simulink model "simulinkDEC"  (R2013b)
settings: Solver=ode45  StartTime=0.0  StopTime=10.0  RelTol=1e-3
undefined symbols (not defined in the file or in its folder): dfilt
libraries: dspsigops x4, dsparch4 x4, dspsrcs4 x1
settings Model: Creator=Johan  LastModifiedBy=Johan

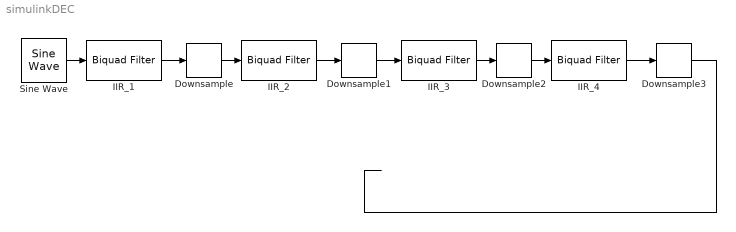
== system simulinkDEC ==
  Downsample{,1..3} (4 alike) : dspsigops/Downsample  N=2  phase=0  RateOptions=Enforce single-rate processing  smode=Allow multirate  fmode=Maintain input frame size  ic=0
  IIR_1 : dsparch4/Biquad Filter  Tag=BlockMethodSubSystem  IIRFiltStruct=Direct form I  CoeffSource=Specify via dialog  BiQuadCoeffs=[1 2 1 1 -1.70675000346131567 0.76497690612845648]  a0Flag=None  IC=0  ICnum=0  ICden=0  denAccumFracLength=30  denProdOutputFracLength=30  secondMemoryFracLength=15  roundingMode=Floor  overflowMode=off  ScaleValues=[0.014556725666785229;1]  optimizeScaleValues=off  ScaleValueMode=Specify via input port (g)  scaleValueFracLength=14  FilterSource=Specify via dialog  dfiltObjectName=dfilt.df2tsos([1 0.3 0.4],[1 0.1 0.2])
  IIR_2 : dsparch4/Biquad Filter  Tag=BlockMethodSubSystem  IIRFiltStruct=Direct form I  CoeffSource=Specify via dialog  BiQuadCoeffs=[1 2 1 1 -1.60151276454445912 0.700754075354693917]  a0Flag=Warning  IC=0  ICnum=0  ICden=0  denAccumFracLength=30  denProdOutputFracLength=30  secondMemoryFracLength=15  roundingMode=Floor  overflowMode=off  ScaleValues=[0.0248103277025586919;0.891250938133745563]  optimizeScaleValues=on  ScaleValueMode=Specify via input port (g)  scaleValueFracLength=14  FilterSource=Specify via dialog  dfiltObjectName=dfilt.df2tsos([1 0.3 0.4],[1 0.1 0.2])
  IIR_3 : dsparch4/Biquad Filter  Tag=BlockMethodSubSystem  IIRFiltStruct=Direct form I  CoeffSource=Specify via dialog  BiQuadCoeffs=[1 2 1 1 -1.29699998625984003 0.553258028437339289]  a0Flag=Warning  IC=0  ICnum=0  ICden=0  denAccumFracLength=30  denProdOutputFracLength=30  secondMemoryFracLength=15  roundingMode=Floor  overflowMode=off  ScaleValues=[0.0640645105443748281;0.891250938133745563]  optimizeScaleValues=on  ScaleValueMode=Specify via input port (g)  scaleValueFracLength=14  FilterSource=Specify via dialog  dfiltObjectName=dfilt.df2tsos([1 0.3 0.4],[1 0.1 0.2])
  IIR_4 : dsparch4/Biquad Filter  Tag=BlockMethodSubSystem  IIRFiltStruct=Direct form I  CoeffSource=Specify via dialog  BiQuadCoeffs=[1 2 1 1 -0.720403563238159794 0.382932497160983876]  a0Flag=Warning  IC=0  ICnum=0  ICden=0  denAccumFracLength=30  denProdOutputFracLength=30  secondMemoryFracLength=15  roundingMode=Floor  overflowMode=off  ScaleValues=[0.165632233480706048;0.891250938133745563]  optimizeScaleValues=on  ScaleValueMode=Specify via input port (g)  scaleValueFracLength=14  FilterSource=Specify via dialog  dfiltObjectName=dfilt.df2tsos([1 0.3 0.4],[1 0.1 0.2])
  Sine Wave : dspsrcs4/Sine Wave  Amplitude=5  Frequency=20000  Phase=0  SampleMode=Discrete  OutComplex=Real  CompMethod=Trigonometric fcn  TableSize=Speed  SampleTime=1/768000  SamplesPerFrame=1  ResetState=Restart at time zero  dataType=double  wordLen=16  udDataType=sfix(16)  fracBitsMode=Best precision  numFracBits=15  OutDataTypeStr=double  LastOutDataTypeStr=double
  wires:
  Sine Wave/1 -> IIR_1/1
  IIR_1/1 -> Downsample/1
  Downsample/1 -> IIR_2/1
  IIR_2/1 -> Downsample1/1
  Downsample1/1 -> IIR_3/1
  IIR_3/1 -> Downsample2/1
  Downsample2/1 -> IIR_4/1
  IIR_4/1 -> Downsample3/1
  Downsample3/1 -> ?
